simulink model "simulink_discrete"  (Simulink 7.7)
settings: Solver=ode45  StartTime=0.0  StopTime=0.5  RelTol=1e-3
undefined symbols (not defined in the file or in its folder): T1, T2
libraries: cstblocks x6
settings Model: Creator=Koldo  LastModifiedBy=Koldo

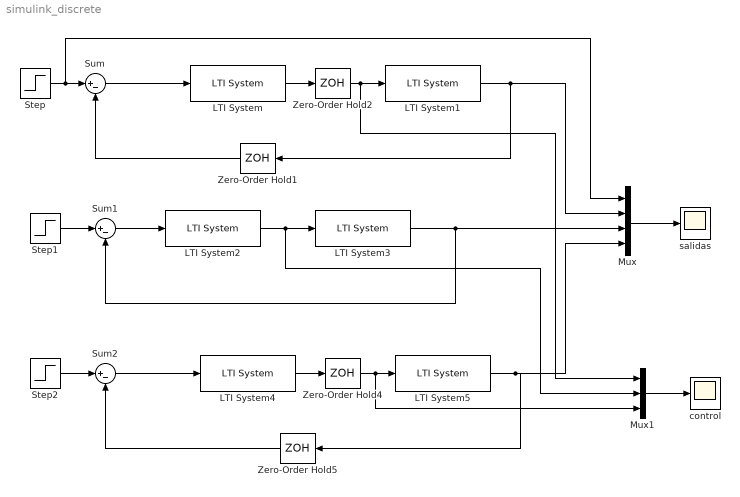
== system simulink_discrete ==
  LTI System : cstblocks/LTI System  SystemSampleTime=-1  sys=CT1_tust  IC=[]
  LTI System1 : cstblocks/LTI System  SystemSampleTime=-1  sys=G  IC=[]
  LTI System2 : cstblocks/LTI System  SystemSampleTime=-1  sys=C  IC=[]
  LTI System3 : cstblocks/LTI System  SystemSampleTime=-1  sys=G  IC=[]
  LTI System4 : cstblocks/LTI System  SystemSampleTime=-1  sys=CT2_tust  IC=[]
  LTI System5 : cstblocks/LTI System  SystemSampleTime=-1  sys=G  IC=[]
  Mux : Mux
  Mux1 : Mux  Inputs=3
  Step : Step  Time=0  SampleTime=0
  Step1 : Step  Time=0  SampleTime=0
  Step2 : Step  Time=0  SampleTime=0
  Sum : Sum  Inputs=|+-
  Sum1 : Sum  Inputs=|+-
  Sum2 : Sum  Inputs=|+-
  Zero-Order Hold1 : ZeroOrderHold  SampleTime=T1
  Zero-Order Hold2 : ZeroOrderHold  SampleTime=T1
  Zero-Order Hold4 : ZeroOrderHold  SampleTime=T2
  Zero-Order Hold5 : ZeroOrderHold  SampleTime=T2
  control : Scope
      settings: MaxDataPoints=50000
  salidas : Scope
      settings: MaxDataPoints=50000
  wires:
  Step/1 -> Sum/1, Mux/1
  Sum/1 -> LTI System/1
  LTI System1/1 -> Mux/2, Zero-Order Hold1/1
  LTI System/1 -> Zero-Order Hold2/1
  Zero-Order Hold2/1 -> LTI System1/1, Mux1/1
  Step1/1 -> Sum1/1
  Sum1/1 -> LTI System2/1
  LTI System3/1 -> Mux/3, Sum1/2
  LTI System2/1 -> LTI System3/1, Mux1/2
  Mux/1 -> salidas/1
  Step2/1 -> Sum2/1
  Sum2/1 -> LTI System4/1
  LTI System5/1 -> Mux/4, Zero-Order Hold5/1
  LTI System4/1 -> Zero-Order Hold4/1
  Zero-Order Hold4/1 -> LTI System5/1, Mux1/3
  Mux1/1 -> control/1
  Zero-Order Hold1/1 -> Sum/2
  Zero-Order Hold5/1 -> Sum2/2
